simulink model "Simulink system"  (R2020a)
settings: Solver=VariableStepAuto  StartTime=0.0  StopTime=1  MaxStep=0.01  RelTol=1e-3
libraries: sldvlib x1
settings Model: Creator=arne-  LastModifiedBy=arne-

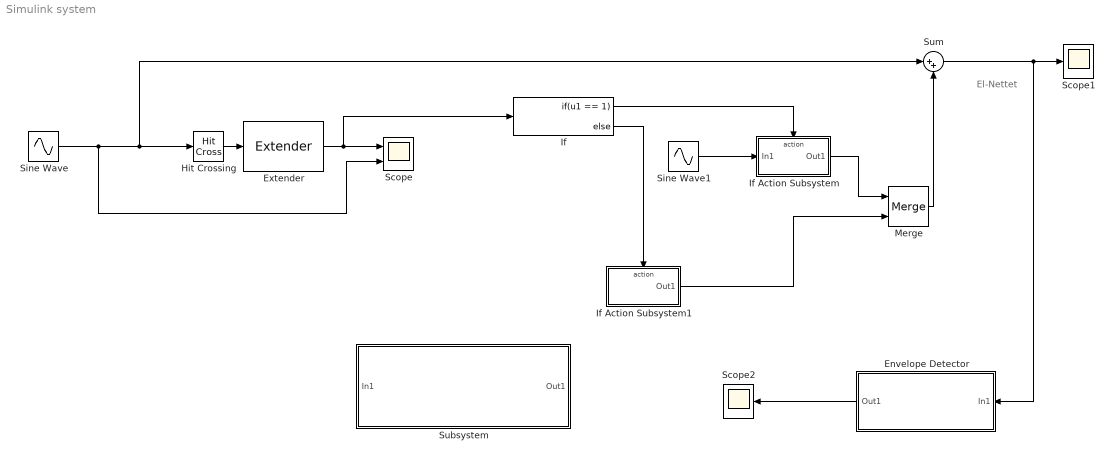
== system Simulink system ==
  note: El-Nettet
  Envelope Detector : Subsystem
  Extender : sldvlib/Temporal Operators/Extender  reset=off  ext_type=Finite  out_hold=5000
      settings: SourceProductBaseCode=SL
  Hit Crossing : HitCross
  If : If  IfExpression=u1 == 1
  If Action Subsystem : Subsystem  TreatAsAtomicUnit=on
  If Action Subsystem1 : Subsystem  TreatAsAtomicUnit=on
  Merge : Merge
  Scope : Scope  NumInputPorts=2
  Scope1 : Scope
  Scope2 : Scope
  Sine Wave : Sin  Amplitude=12.7  Frequency=314.16  SampleTime=0
  Sine Wave1 : Sin  Amplitude=2.5  Frequency=753982.236  SampleTime=0
  Subsystem : Subsystem
  Sum : Sum  Inputs=|++
  wires:
  Hit Crossing/1 -> Extender/1
  Sine Wave/1 -> Scope/2, Sum/1, Hit Crossing/1
  If/1 -> If Action Subsystem/Action
  If/2 -> If Action Subsystem1/Action
  Sine Wave1/1 -> If Action Subsystem/1(In1)
  Merge/1 -> Sum/2
  If Action Subsystem/1(Out1) -> Merge/1
  If Action Subsystem1/1(Out1) -> Merge/2
  Extender/1 -> If/1, Scope/1
  Sum/1 -> Envelope Detector/1(In1), Scope1/1
  Envelope Detector/1(Out1) -> Scope2/1

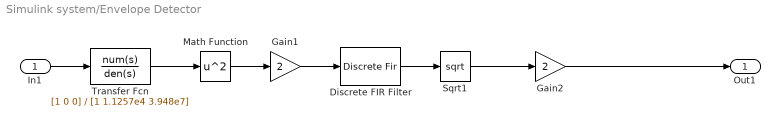
== system Simulink system/Envelope Detector ==
  In1 : Inport
  Discrete FIR Filter : DiscreteFir  Coefficients=1/1000.*ones(1, 1000)  SampleTime=2e-7
  Gain1 : Gain  Gain=2
  Gain2 : Gain  Gain=2
  Math Function : Math  Operator=square  SaturateOnIntegerOverflow=on
  Sqrt1 : Sqrt  SaturateOnIntegerOverflow=on
  Transfer Fcn : TransferFcn  Numerator=[1 0 0]  Denominator=[1 1.1257e4 3.948e7]
  Out1 : Outport
  wires:
  In1/1 -> Transfer Fcn/1
  Transfer Fcn/1 -> Math Function/1
  Math Function/1 -> Gain1/1
  Gain1/1 -> Discrete FIR Filter/1
  Discrete FIR Filter/1 -> Sqrt1/1
  Sqrt1/1 -> Gain2/1
  Gain2/1 -> Out1/1

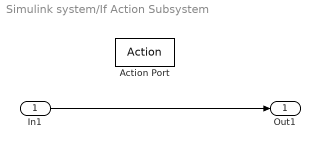
== system Simulink system/If Action Subsystem ==
  In1 : Inport
  Action Port : ActionPort  ActionPortLabel=if(u1 == 1)
  Out1 : Outport
  wires:
  In1/1 -> Out1/1

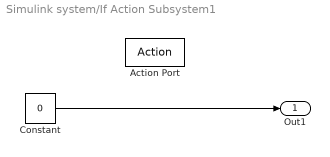
== system Simulink system/If Action Subsystem1 ==
  Action Port : ActionPort  ActionPortLabel=else
  Constant : Constant  Value=0
  Out1 : Outport
  wires:
  Constant/1 -> Out1/1

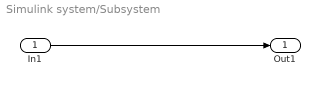
== system Simulink system/Subsystem ==
  In1 : Inport
  Out1 : Outport
  wires:
  In1/1 -> Out1/1
